simulink model "warplab_mimo_4x4"  (Simulink 6.5)
settings: Solver=ode45  StartTime=0.0  StopTime=20000  RelTol=1e-3
undefined symbols (not defined in the file): gcbh, xlBlockLoadCallback
libraries: xbsIndex_r4 x188
(part 10 of 17)

== system warplab_mimo_4x4/Mem_Control/S-R_Latch (Reverse) ==
  S : Inport
  R : Inport  Port=2
  Convert : S-Function  LoadFcn=xlBlockLoadCallback(gcbh);  FunctionName=sysgen  Parameters=ptable_  mask(Xilinx Type Converter Block){infoedit=Hardware notes: rounding and saturating require hardware resources; truncating and wrapping do not., arith_type_sgadvanced=, arith_type=Boolean, n_bits=16, bin_pt=14, quantization_sgadvanced=, quantization=Truncate, overflow_sgadvanced=, overflow=Wrap, latency=0, dbl_ovrd_sgadvanced=, dbl_ovrd=off, pipeline_sgadvanced=, pipeline=off, xl_use_area_sgadvanced=, xl_use_area=off, xl_area=[0,0,0,0,0,0,0], has_advanced_control=0, sggui_pos=20,20,374,375, block_type=convert, block_version=8.2, sg_icon_stat=30,14,1,1,white,blue,0,0eb6e735, sg_mask_display=|, sg_list_contents=, sg_blockgui_xml=}
      mask sg_mask_display=|
      | fprintf('','COMMENT: begin icon graphics');
      | patch([0 30 30 0 ],[0 0 14 14 ],[0.77 0.82 0.91]);
      | patch([11 9 12 9 11 15 16 17 21 18 15 13 16 13 15 18 21 17 16 15 11 ],[2 4 7 10 12 12 11 12 12 9 12 10 7 4 2 5 2 2 3 2 2 ],[0.98 0.96 0.92]);
      | plot([0 0 30 30 0 ],[0 14 14 0 0 ]);
      | fprintf('','COMMENT: end icon graphics');
      | fprintf('','COMMENT: begin icon text');
      | color('black');port_label('output',1,'cast');
      | fprintf('','COMMENT: end icon text');
      mask prompts: infoedit ""; arith_type_sgadvanced ""; arith_type "Type"; n_bits "Number of bits"; bin_pt "Binary point"; quantization_sgadvanced ""; overflow_sgadvanced ""; dbl_ovrd_sgadvanced ""; dbl_ovrd "Override with doubles"; pipeline_sgadvanced ""; pipeline "Pipeline for maximum performance"; xl_use_area_sgadvanced ""; xl_use_area "Define FPGA area for resource estimation"; xl_area "FPGA area [slices, FFs, BRAMs, LUTs, IOBs, emb. mults, TBUFs]"; has_advanced_control ""; sggui_pos ""; block_type ""; block_version ""; sg_icon_stat ""; sg_mask_display ""; sg_list_contents ""; sg_blockgui_xml ""
      mask help: Hardware notes: rounding and saturating require hardware resources; truncating and wrapping do not.
      mask init: same as warplab_mimo_4x4/Mem_Control/Convert1
      settings: CopyFcn=xlBlockMoveCallback(gcbh);  DeleteFcn=xlDestroyGui(gcbh);  ModelCloseFcn=xlDestroyGui(gcbh);  PreSaveFcn=xlBlockPreSaveCallback(gcbh);  PostSaveFcn=xlBlockPostSaveCallback(gcbh);  DestroyFcn=xlDestroyGui(gcbh);  OpenFcn=xlOpenGui(gcbh, 'convert_gui.xml', @convertenablement, -1)  CloseFcn=xlDestroyGui(gcbh);  MoveFcn=xlBlockMoveCallback(gcbh);
      mask Help: eval('xlWeb(xlhtmldoclink(''Convert''))');
      mask StyleString: edit,edit,popup(Boolean|Signed  (2's comp)|Unsigned),edit,edit,edit,popup(Truncate|Round  (unbiased: +/- Inf)|Round  (unbiased: Even Values)),edit,popup(Wrap|Saturate|Flag as error),edit,edit,checkbox,edit,checkbox,edit,checkbox,edit,edit,edit,edit,edit,edit,edit,edit,edit
      mask Display:
      | fprintf('','COMMENT: begin icon graphics');
      | patch([0 30 30 0 ],[0 0 14 14 ],[0.77 0.82 0.91]);
      | patch([11 9 12 9 11 15 16 17 21 18 15 13 16 13 15 18 21 17 16 15 11 ],[2 4 7 10 12 12 11 12 12 9 12 10 7 4 2 5 2 2 3 2 2 ],[0.98 0.96 0.92]);
      | plot([0 0 30 30 0 ],[0 14 14 0 0 ]);
      | fprintf('','COMMENT: end icon graphics');
      | fprintf('','COMMENT: begin icon text');
      | color('black');port_label('output',1,'cast');
      | fprintf('','COMMENT: end icon text');
  Convert1 : S-Function  LoadFcn=xlBlockLoadCallback(gcbh);  FunctionName=sysgen  Parameters=ptable_  mask(Xilinx Type Converter Block){infoedit=Hardware notes: rounding and saturating require hardware resources; truncating and wrapping do not., arith_type_sgadvanced=, arith_type=Boolean, n_bits=16, bin_pt=14, quantization_sgadvanced=, quantization=Truncate, overflow_sgadvanced=, overflow=Wrap, latency=0, dbl_ovrd_sgadvanced=, dbl_ovrd=off, pipeline_sgadvanced=, pipeline=off, xl_use_area_sgadvanced=, xl_use_area=off, xl_area=[0,0,0,0,0,0,0], has_advanced_control=0, sggui_pos=20,20,374,375, block_type=convert, block_version=8.2, sg_icon_stat=30,14,1,1,white,blue,0,0eb6e735, sg_mask_display=|, sg_list_contents=, sg_blockgui_xml=}
      mask sg_mask_display=|
      | fprintf('','COMMENT: begin icon graphics');
      | patch([0 30 30 0 ],[0 0 14 14 ],[0.77 0.82 0.91]);
      | patch([11 9 12 9 11 15 16 17 21 18 15 13 16 13 15 18 21 17 16 15 11 ],[2 4 7 10 12 12 11 12 12 9 12 10 7 4 2 5 2 2 3 2 2 ],[0.98 0.96 0.92]);
      | plot([0 0 30 30 0 ],[0 14 14 0 0 ]);
      | fprintf('','COMMENT: end icon graphics');
      | fprintf('','COMMENT: begin icon text');
      | color('black');port_label('output',1,'cast');
      | fprintf('','COMMENT: end icon text');
      mask prompts: infoedit ""; arith_type_sgadvanced ""; arith_type "Type"; n_bits "Number of bits"; bin_pt "Binary point"; quantization_sgadvanced ""; overflow_sgadvanced ""; dbl_ovrd_sgadvanced ""; dbl_ovrd "Override with doubles"; pipeline_sgadvanced ""; pipeline "Pipeline for maximum performance"; xl_use_area_sgadvanced ""; xl_use_area "Define FPGA area for resource estimation"; xl_area "FPGA area [slices, FFs, BRAMs, LUTs, IOBs, emb. mults, TBUFs]"; has_advanced_control ""; sggui_pos ""; block_type ""; block_version ""; sg_icon_stat ""; sg_mask_display ""; sg_list_contents ""; sg_blockgui_xml ""
      mask help: Hardware notes: rounding and saturating require hardware resources; truncating and wrapping do not.
      mask init: same as warplab_mimo_4x4/Mem_Control/Convert1
      settings: CopyFcn=xlBlockMoveCallback(gcbh);  DeleteFcn=xlDestroyGui(gcbh);  ModelCloseFcn=xlDestroyGui(gcbh);  PreSaveFcn=xlBlockPreSaveCallback(gcbh);  PostSaveFcn=xlBlockPostSaveCallback(gcbh);  DestroyFcn=xlDestroyGui(gcbh);  OpenFcn=xlOpenGui(gcbh, 'convert_gui.xml', @convertenablement, -1)  CloseFcn=xlDestroyGui(gcbh);  MoveFcn=xlBlockMoveCallback(gcbh);
      mask Help: eval('xlWeb(xlhtmldoclink(''Convert''))');
      mask StyleString: edit,edit,popup(Boolean|Signed  (2's comp)|Unsigned),edit,edit,edit,popup(Truncate|Round  (unbiased: +/- Inf)|Round  (unbiased: Even Values)),edit,popup(Wrap|Saturate|Flag as error),edit,edit,checkbox,edit,checkbox,edit,checkbox,edit,edit,edit,edit,edit,edit,edit,edit,edit
      mask Display:
      | fprintf('','COMMENT: begin icon graphics');
      | patch([0 30 30 0 ],[0 0 14 14 ],[0.77 0.82 0.91]);
      | patch([11 9 12 9 11 15 16 17 21 18 15 13 16 13 15 18 21 17 16 15 11 ],[2 4 7 10 12 12 11 12 12 9 12 10 7 4 2 5 2 2 3 2 2 ],[0.98 0.96 0.92]);
      | plot([0 0 30 30 0 ],[0 14 14 0 0 ]);
      | fprintf('','COMMENT: end icon graphics');
      | fprintf('','COMMENT: begin icon text');
      | color('black');port_label('output',1,'cast');
      | fprintf('','COMMENT: end icon text');
  Register : S-Function  LoadFcn=xlBlockLoadCallback(gcbh);  FunctionName=sysgen  Parameters=ptable_  mask(Xilinx Register Block){init=1, rst_sgadvanced=, rst=on, en_sgadvanced=, en=on, dbl_ovrd_sgadvanced=, dbl_ovrd=off, xl_use_area_sgadvanced=, xl_use_area=off, xl_area=[0,0,0,0,0,0,0], has_advanced_control=0, sggui_pos=-1,-1,-1,-1, block_type=register, block_version=8.2, sg_icon_stat=50,64,3,1,white,blue,0,923c1847, sg_mask_display=|, sg_list_contents=, sg_blockgui_xml=}
      mask sg_mask_display=|
      | fprintf('','COMMENT: begin icon graphics');
      | patch([0 50 50 0 ],[0 0 64 64 ],[0.77 0.82 0.91]);
      | patch([11 3 15 3 11 24 28 32 46 35 24 16 28 16 24 35 46 32 28 24 11 ],[12 20 32 44 52 52 48 52 52 41 52 44 32 20 12 23 12 12 16 12 12 ],[0.98 0.96 0.92]);
      | plot([0 0 50 50 0 ],[0 64 64 0 0 ]);
      | fprintf('','COMMENT: end icon graphics');
      | fprintf('','COMMENT: begin icon text');
      | color('black');port_label('input',1,'d');
      | color('black');port_label('input',2,'rst');
      | color('black');port_label('input',3,'en');
      | color('black');port_label('output',1,'q');
      | color('black');disp('\bf{z^{-1}}','texmode','on');
      | fprintf('','COMMENT: end icon text');
      mask prompts: init "Initial value"; rst_sgadvanced ""; rst "Provide synchronous reset port"; en_sgadvanced ""; en "Provide enable port"; dbl_ovrd_sgadvanced ""; dbl_ovrd "Override with doubles"; xl_use_area_sgadvanced ""; xl_use_area "Define FPGA area for resource estimation"; xl_area "FPGA area [slices, FFs, BRAMs, LUTs, IOBs, emb. mults, TBUFs]"; has_advanced_control ""; sggui_pos ""; block_type ""; block_version ""; sg_icon_stat ""; sg_mask_display ""; sg_list_contents ""; sg_blockgui_xml ""
      mask help: Xilinx Register
      mask init: same as warplab_mimo_4x4/Mem_Control/Register
      settings: CopyFcn=xlBlockMoveCallback(gcbh);  DeleteFcn=xlDestroyGui(gcbh);  ModelCloseFcn=xlDestroyGui(gcbh);  PreSaveFcn=xlBlockPreSaveCallback(gcbh);  PostSaveFcn=xlBlockPostSaveCallback(gcbh);  DestroyFcn=xlDestroyGui(gcbh);  OpenFcn=xlOpenGui(gcbh, 'register_gui.xml', @xlmagicenablement, -1)  CloseFcn=xlDestroyGui(gcbh);  MoveFcn=xlBlockMoveCallback(gcbh);
      mask Help: eval('xlWeb(xlhtmldoclink(''Register''))');
      mask Display:
      | fprintf('','COMMENT: begin icon graphics');
      | patch([0 50 50 0 ],[0 0 64 64 ],[0.77 0.82 0.91]);
      | patch([11 3 15 3 11 24 28 32 46 35 24 16 28 16 24 35 46 32 28 24 11 ],[12 20 32 44 52 52 48 52 52 41 52 44 32 20 12 23 12 12 16 12 12 ],[0.98 0.96 0.92]);
      | plot([0 0 50 50 0 ],[0 64 64 0 0 ]);
      | fprintf('','COMMENT: end icon graphics');
      | fprintf('','COMMENT: begin icon text');
      | color('black');port_label('input',1,'d');
      | color('black');port_label('input',2,'rst');
      | color('black');port_label('input',3,'en');
      | color('black');port_label('output',1,'q');
      | color('black');disp('\bf{z^{-1}}','texmode','on');
      | fprintf('','COMMENT: end icon text');
  zero3 : S-Function  LoadFcn=xlBlockLoadCallback(gcbh);  FunctionName=sysgen  Parameters=ptable_  mask(Xilinx Constant Block Block){arith_type_sgadvanced=, arith_type=Boolean, const=0, n_bits=1, bin_pt=0, explicit_period_sgadvanced=, explicit_period=off, period=1, dsp48_infoedit=The use of this block for DSP48 instructions is deprecated.  Please use the Opmode block., equ=P=C, opselect_sgadvanced=, opselect=C, inp2_sgadvanced=, inp2=PCIN>>17, opr_sgadvanced=, opr=+, inp1_sgadvanced=, inp1=P, carry_sgadvanced=, carry=CIN, dbl_ovrd_sgadvanced=, dbl_ovrd=off, has_advanced_control=0, sggui_pos=-1,-1,-1,-1, block_type=constant, block_version=VER_STRING_GOES_HERE, sg_icon_stat=20,18,0,1,white,blue,0,c7c04a0c, sg_mask_display=|, sg_list_contents=, sg_blockgui_xml=}
      mask sg_mask_display=|
      | fprintf('','COMMENT: begin icon graphics');
      | patch([0 55 55 0 ],[0 0 26 26 ],[0.77 0.82 0.91]);
      | patch([20 16 22 16 20 27 29 31 38 32 26 22 28 22 26 32 38 31 29 27 20 ],[3 7 13 19 23 23 21 23 23 17 23 19 13 7 3 9 3 3 5 3 3 ],[0.98 0.96 0.92]);
      | plot([0 0 55 55 0 ],[0 26 26 0 0 ]);
      | fprintf('','COMMENT: end icon graphics');
      | fprintf('','COMMENT: begin icon text');
      | color('black');port_label('output',1,'0');
      | fprintf('','COMMENT: end icon text');
      mask prompts: arith_type_sgadvanced ""; arith_type "Type"; const "Constant value"; n_bits "Number of bits"; bin_pt "Binary point"; explicit_period_sgadvanced ""; explicit_period "Sampled constant"; period "Sample period"; dsp48_infoedit ""; equ "DSP48 operation"; opselect_sgadvanced ""; opselect "Operation select"; inp2_sgadvanced ""; inp2 "Z mux"; opr_sgadvanced ""; opr "Operand"; inp1_sgadvanced ""; inp1 "YX muxes"; carry_sgadvanced ""; carry "Carry input"; dbl_ovrd_sgadvanced ""; dbl_ovrd "Override with doubles"; has_advanced_control ""; sggui_pos ""; block_type ""; block_version ""; sg_icon_stat ""; sg_mask_display ""; sg_list_contents ""; sg_blockgui_xml ""
      mask help: Xilinx Constant Block
      mask init: same as warplab_mimo_4x4/CaptureDone/zero3
      settings: CopyFcn=xlBlockMoveCallback(gcbh);  DeleteFcn=xlDestroyGui(gcbh);  ModelCloseFcn=xlDestroyGui(gcbh);  PreSaveFcn=xlBlockPreSaveCallback(gcbh);  PostSaveFcn=xlBlockPostSaveCallback(gcbh);  DestroyFcn=xlDestroyGui(gcbh);  OpenFcn=xlOpenGui(gcbh, 'constant_gui.xml', @constantenablement, @constantaction)  CloseFcn=xlDestroyGui(gcbh);  MoveFcn=xlBlockMoveCallback(gcbh);
      mask Help: eval('xlWeb(xlhtmldoclink(''Constant''))');
      mask StyleString: edit,popup(Boolean|Signed (2's comp)|Unsigned|DSP48 Instruction),edit,edit,edit,edit,checkbox,edit,edit,edit,edit,popup(C + A*B|PCIN + A*B|P + A*B|A * B|C + A:B|C - A:B|C|Custom),edit,popup(0|PCIN|P|C|PCIN>>17|P>>17),edit,popup(+|-),edit,popup(0|P|A:B|A*B|C|P+C|A:B+C),edit,popup(0|1|CIN|~SIGN(P or PCIN)|~SIGN(A*B or A:B)|~SIGND(A*B or A:B)),edit,checkbox,edit,edit,edit,edit,edit,edit,edit,edit
      mask Display:
      | fprintf('','COMMENT: begin icon graphics');
      | patch([0 55 55 0 ],[0 0 26 26 ],[0.77 0.82 0.91]);
      | patch([20 16 22 16 20 27 29 31 38 32 26 22 28 22 26 32 38 31 29 27 20 ],[3 7 13 19 23 23 21 23 23 17 23 19 13 7 3 9 3 3 5 3 3 ],[0.98 0.96 0.92]);
      | plot([0 0 55 55 0 ],[0 26 26 0 0 ]);
      | fprintf('','COMMENT: end icon graphics');
      | fprintf('','COMMENT: begin icon text');
      | color('black');port_label('output',1,'0');
      | fprintf('','COMMENT: end icon text');
  Q : Outport
  wires:
  zero3/1 -> Register/1
  S/1 -> Convert/1
  R/1 -> Convert1/1
  Register/1 -> Q/1
  Convert/1 -> Register/2
  Convert1/1 -> Register/3

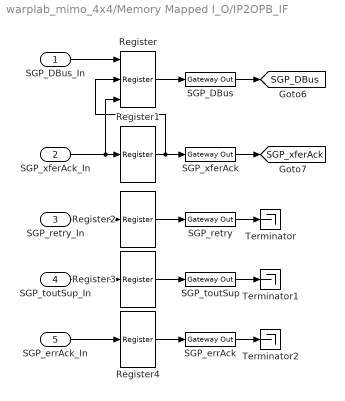
== system warplab_mimo_4x4/Memory Mapped I_O/IP2OPB_IF ==
  SGP_DBus_In : Inport
  SGP_xferAck_In : Inport  Port=2
  SGP_retry_In : Inport  Port=3
  SGP_toutSup_In : Inport  Port=4
  SGP_errAck_In : Inport  Port=5
  Register : xbsIndex_r4/Register  init=0  rst=on  en=on  dbl_ovrd=off  block_type=register
      settings: xl_area=[0, 0, 0, 0, 0, 0, 0]  block_version=VER_STRING_GOES_HERE
  Register{1..4} (4 alike) : xbsIndex_r4/Register  init=0  rst=off  en=off  dbl_ovrd=off  block_type=register
      settings: xl_area=[0, 0, 0, 0, 0, 0, 0]  block_version=VER_STRING_GOES_HERE
  SGP_DBus : xbsIndex_r4/Gateway Out  hdl_port=on  timing_constraint=None  locs_specified=off  LOCs={}  block_type=gatewayout
      settings: infoedit="Gateway out block.  Converts Xilinx fixed point inputs into ouputs of type Simulink integer, double, or fixed point.<P><P>Hardware notes:  In hardware these blocks become top level output ports or are discarded, depending on how they are configured."  xl_area=[0, 0, 0, 0, 0, 0, 0]  block_version=VER_STRING_GOES_HERE
  SGP_errAck : xbsIndex_r4/Gateway Out  hdl_port=on  timing_constraint=None  locs_specified=off  LOCs={}  block_type=gatewayout
      settings: infoedit="Gateway out block.  Converts Xilinx fixed point inputs into ouputs of type Simulink integer, double, or fixed point.<P><P>Hardware notes:  In hardware these blocks become top level output ports or are discarded, depending on how they are configured."  xl_area=[0, 0, 0, 0, 0, 0, 0]  block_version=VER_STRING_GOES_HERE
  SGP_retry : xbsIndex_r4/Gateway Out  hdl_port=on  timing_constraint=None  locs_specified=off  LOCs={}  block_type=gatewayout
      settings: infoedit="Gateway out block.  Converts Xilinx fixed point inputs into ouputs of type Simulink integer, double, or fixed point.<P><P>Hardware notes:  In hardware these blocks become top level output ports or are discarded, depending on how they are configured."  xl_area=[0, 0, 0, 0, 0, 0, 0]  block_version=VER_STRING_GOES_HERE
  SGP_toutSup : xbsIndex_r4/Gateway Out  hdl_port=on  timing_constraint=None  locs_specified=off  LOCs={}  block_type=gatewayout
      settings: infoedit="Gateway out block.  Converts Xilinx fixed point inputs into ouputs of type Simulink integer, double, or fixed point.<P><P>Hardware notes:  In hardware these blocks become top level output ports or are discarded, depending on how they are configured."  xl_area=[0, 0, 0, 0, 0, 0, 0]  block_version=VER_STRING_GOES_HERE
  SGP_xferAck : xbsIndex_r4/Gateway Out  hdl_port=on  timing_constraint=None  locs_specified=off  LOCs={}  block_type=gatewayout
      settings: infoedit="Gateway out block.  Converts Xilinx fixed point inputs into ouputs of type Simulink integer, double, or fixed point.<P><P>Hardware notes:  In hardware these blocks become top level output ports or are discarded, depending on how they are configured."  xl_area=[0, 0, 0, 0, 0, 0, 0]  block_version=VER_STRING_GOES_HERE
  Terminator : Terminator
  Terminator1 : Terminator
  Terminator2 : Terminator
  tag scope: SGP_DBus=global, SGP_xferAck=global
  wires:
  SGP_errAck/1 -> Terminator2/1
  SGP_toutSup/1 -> Terminator1/1
  SGP_retry/1 -> Terminator/1
  Register1/1 -> Register/2, SGP_xferAck/1
  SGP_errAck_In/1 -> Register4/1
  SGP_toutSup_In/1 -> Register3/1
  SGP_retry_In/1 -> Register2/1
  SGP_xferAck_In/1 -> Register1/1, Register/3
  SGP_DBus_In/1 -> Register/1
  SGP_DBus/1 -> [SGP_DBus]
  SGP_xferAck/1 -> [SGP_xferAck]
  Register2/1 -> SGP_retry/1
  Register3/1 -> SGP_toutSup/1
  Register4/1 -> SGP_errAck/1
  Register/1 -> SGP_DBus/1

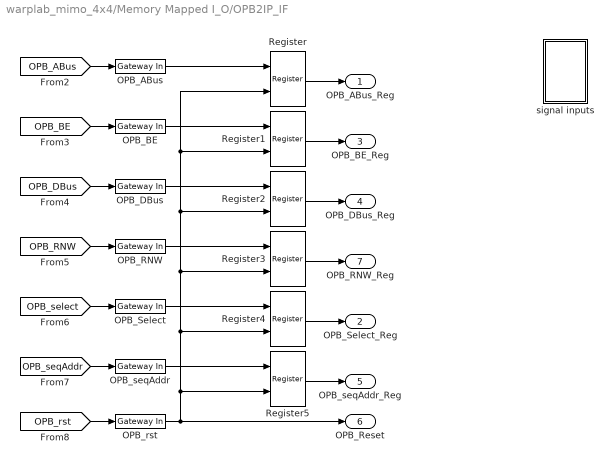
== system warplab_mimo_4x4/Memory Mapped I_O/OPB2IP_IF ==
  OPB_ABus : xbsIndex_r4/Gateway In  arith_type=Unsigned  n_bits=32  bin_pt=0  quantization="Round  (unbiased: +/- Inf)"  overflow=Saturate  period=1  dbl_ovrd=off  timing_constraint=None  locs_specified=off  LOCs={}  block_type=gatewayin
      settings: infoedit="Gateway in block.  Converts inputs of type Simulink integer, double and fixed point to  Xilinx fixed point type.<P><P>Hardware notes:  In hardware these blocks become top level input ports."  xl_area=[0, 0, 0, 0, 0, 0, 0]  block_version=VER_STRING_GOES_HERE
  OPB_BE : xbsIndex_r4/Gateway In  arith_type=Unsigned  n_bits=4  bin_pt=0  quantization="Round  (unbiased: +/- Inf)"  overflow=Saturate  period=1  dbl_ovrd=off  timing_constraint=None  locs_specified=off  LOCs={}  block_type=gatewayin
      settings: infoedit="Gateway in block.  Converts inputs of type Simulink integer, double and fixed point to  Xilinx fixed point type.<P><P>Hardware notes:  In hardware these blocks become top level input ports."  xl_area=[0, 0, 0, 0, 0, 0, 0]  block_version=VER_STRING_GOES_HERE
  OPB_DBus : xbsIndex_r4/Gateway In  arith_type=Unsigned  n_bits=32  bin_pt=0  quantization="Round  (unbiased: +/- Inf)"  overflow=Saturate  period=1  dbl_ovrd=off  timing_constraint=None  locs_specified=off  LOCs={}  block_type=gatewayin
      settings: infoedit="Gateway in block.  Converts inputs of type Simulink integer, double and fixed point to  Xilinx fixed point type.<P><P>Hardware notes:  In hardware these blocks become top level input ports."  xl_area=[0, 0, 0, 0, 0, 0, 0]  block_version=VER_STRING_GOES_HERE
  OPB_RNW : xbsIndex_r4/Gateway In  arith_type=Boolean  n_bits=1  bin_pt=0  quantization="Round  (unbiased: +/- Inf)"  overflow=Saturate  period=1  dbl_ovrd=off  timing_constraint=None  locs_specified=off  LOCs={}  block_type=gatewayin
      settings: infoedit="Gateway in block.  Converts inputs of type Simulink integer, double and fixed point to  Xilinx fixed point type.<P><P>Hardware notes:  In hardware these blocks become top level input ports."  xl_area=[0, 0, 0, 0, 0, 0, 0]  block_version=VER_STRING_GOES_HERE
  OPB_Select : xbsIndex_r4/Gateway In  arith_type=Boolean  n_bits=1  bin_pt=0  quantization="Round  (unbiased: +/- Inf)"  overflow=Saturate  period=1  dbl_ovrd=off  timing_constraint=None  locs_specified=off  LOCs={}  block_type=gatewayin
      settings: infoedit="Gateway in block.  Converts inputs of type Simulink integer, double and fixed point to  Xilinx fixed point type.<P><P>Hardware notes:  In hardware these blocks become top level input ports."  xl_area=[0, 0, 0, 0, 0, 0, 0]  block_version=VER_STRING_GOES_HERE
  OPB_rst : xbsIndex_r4/Gateway In  arith_type=Boolean  n_bits=1  bin_pt=0  quantization="Round  (unbiased: +/- Inf)"  overflow=Saturate  period=1  dbl_ovrd=off  timing_constraint=None  locs_specified=off  LOCs={}  block_type=gatewayin
      settings: infoedit="Gateway in block.  Converts inputs of type Simulink integer, double and fixed point to  Xilinx fixed point type.<P><P>Hardware notes:  In hardware these blocks become top level input ports."  xl_area=[0, 0, 0, 0, 0, 0, 0]  block_version=VER_STRING_GOES_HERE
  OPB_seqAddr : xbsIndex_r4/Gateway In  arith_type=Boolean  n_bits=1  bin_pt=0  quantization="Round  (unbiased: +/- Inf)"  overflow=Saturate  period=1  dbl_ovrd=off  timing_constraint=None  locs_specified=off  LOCs={}  block_type=gatewayin
      settings: infoedit="Gateway in block.  Converts inputs of type Simulink integer, double and fixed point to  Xilinx fixed point type.<P><P>Hardware notes:  In hardware these blocks become top level input ports."  xl_area=[0, 0, 0, 0, 0, 0, 0]  block_version=VER_STRING_GOES_HERE
  Register{,1..5} (6 alike) : xbsIndex_r4/Register  init=0  rst=on  en=off  dbl_ovrd=off  block_type=register
      settings: xl_area=[0, 0, 0, 0, 0, 0, 0]  block_version=VER_STRING_GOES_HERE
  signal inputs : Subsystem
  OPB_ABus_Reg : Outport
  OPB_Select_Reg : Outport  Port=2
  OPB_BE_Reg : Outport  Port=3
  OPB_DBus_Reg : Outport  Port=4
  OPB_seqAddr_Reg : Outport  Port=5
  OPB_Reset : Outport  Port=6
  OPB_RNW_Reg : Outport  Port=7
  wires:
  Register4/1 -> OPB_Select_Reg/1
  OPB_Select/1 -> Register4/1
  OPB_BE/1 -> Register1/1
  OPB_ABus/1 -> Register/1
  [OPB_select] -> OPB_Select/1
  [OPB_seqAddr] -> OPB_seqAddr/1
  [OPB_rst] -> OPB_rst/1
  [OPB_RNW] -> OPB_RNW/1
  [OPB_DBus] -> OPB_DBus/1
  [OPB_BE] -> OPB_BE/1
  [OPB_ABus] -> OPB_ABus/1
  Register/1 -> OPB_ABus_Reg/1
  OPB_rst/1 -> Register4/2, Register1/2, Register/2, Register2/2, Register3/2, Register5/2, OPB_Reset/1
  Register5/1 -> OPB_seqAddr_Reg/1
  Register3/1 -> OPB_RNW_Reg/1
  Register2/1 -> OPB_DBus_Reg/1
  Register1/1 -> OPB_BE_Reg/1
  OPB_seqAddr/1 -> Register5/1
  OPB_RNW/1 -> Register3/1
  OPB_DBus/1 -> Register2/1

== system warplab_mimo_4x4/Memory Mapped I_O/ack_gen ==
  ps : Inport
  rst : Inport  Port=2
  Inverter1 : xbsIndex_r4/Inverter  en=off  latency=0  dbl_ovrd=off  block_type=inv
      settings: xl_area=[0, 0, 0, 0, 0, 0, 0]  block_version=VER_STRING_GOES_HERE
  Inverter2 : xbsIndex_r4/Inverter  en=off  latency=0  dbl_ovrd=off  block_type=inv
      settings: xl_area=[0, 0, 0, 0, 0, 0, 0]  block_version=VER_STRING_GOES_HERE
  Logical : xbsIndex_r4/Logical  logical_function=AND  inputs=3  en=off  latency=0  precision=Full  arith_type=Unsigned  n_bits=8  bin_pt=2  align_bp=on  dbl_ovrd=off  block_type=logical
      settings: xl_area=[0, 0, 0, 0, 0, 0, 0]  block_version=VER_STRING_GOES_HERE
  Register : xbsIndex_r4/Register  init=0  rst=off  en=off  dbl_ovrd=off  block_type=register
      settings: xl_area=[0, 0, 0, 0, 0, 0, 0]  block_version=VER_STRING_GOES_HERE
  ack : Outport
  wires:
  Logical/1 -> ack/1
  rst/1 -> Inverter1/1
  Inverter1/1 -> Logical/3
  Register/1 -> Inverter2/1
  Inverter2/1 -> Logical/2
  ps/1 -> Register/1, Logical/1

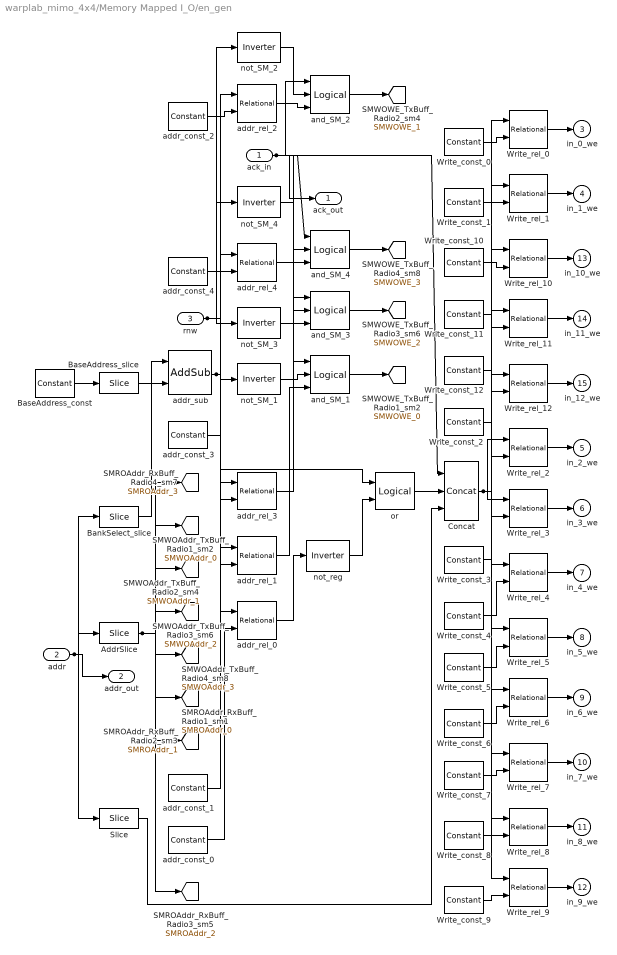
== system warplab_mimo_4x4/Memory Mapped I_O/en_gen ==
  ack_in : Inport
  addr : Inport  Port=2
  rnw : Inport  Port=3
  AddrSlice : xbsIndex_r4/Slice  nbits=14  boolean_output=off  mode=Lower Bit Location + Width  bit1=0  base1=MSB of Input  bit0=2  base0=LSB of Input  dbl_ovrd=off  block_type=slice
      settings: infoedit="Extracts a given range of bits from each input sample and presents it at the output.  The output type is ordinarily unsigned with binary point at zero, but can be Boolean when the slice is one bit wide.<P><P>Hardware notes: In hardware this block costs nothing."  block_version=VER_STRING_GOES_HERE
  BankSelect_slice : xbsIndex_r4/Slice  nbits=4  boolean_output=off  mode=Lower Bit Location + Width  bit1=0  base1=MSB of Input  bit0=16  base0=LSB of Input  dbl_ovrd=off  block_type=slice
      settings: infoedit="Extracts a given range of bits from each input sample and presents it at the output.  The output type is ordinarily unsigned with binary point at zero, but can be Boolean when the slice is one bit wide.<P><P>Hardware notes: In hardware this block costs nothing."  block_version=VER_STRING_GOES_HERE
  BaseAddress_const : xbsIndex_r4/Constant  arith_type=Unsigned  const=0  n_bits=32  bin_pt=0  explicit_period=off  period=1  equ=P=C  opselect=C  inp2=PCIN>>17  opr=+  inp1=P  carry=CIN  dbl_ovrd=off  block_type=constant
      settings: block_version=VER_STRING_GOES_HERE
  BaseAddress_slice : xbsIndex_r4/Slice  nbits=4  boolean_output=off  mode=Lower Bit Location + Width  bit1=0  base1=MSB of Input  bit0=16  base0=LSB of Input  dbl_ovrd=off  block_type=slice
      settings: infoedit="Extracts a given range of bits from each input sample and presents it at the output.  The output type is ordinarily unsigned with binary point at zero, but can be Boolean when the slice is one bit wide.<P><P>Hardware notes: In hardware this block costs nothing."  block_version=VER_STRING_GOES_HERE
  Concat : xbsIndex_r4/Concat  num_inputs=3  dbl_ovrd=off  block_type=concat
      settings: block_version=VER_STRING_GOES_HERE
  Slice : xbsIndex_r4/Slice  nbits=4  boolean_output=off  mode=Lower Bit Location + Width  bit1=0  base1=MSB of Input  bit0=2  base0=LSB of Input  dbl_ovrd=off  block_type=slice
      settings: infoedit="Extracts a given range of bits from each input sample and presents it at the output.  The output type is ordinarily unsigned with binary point at zero, but can be Boolean when the slice is one bit wide.<P><P>Hardware notes: In hardware this block costs nothing."  block_version=VER_STRING_GOES_HERE
  Write_const_0 : xbsIndex_r4/Constant  arith_type=Unsigned  const=32  n_bits=6  bin_pt=0  explicit_period=off  period=1  equ=P=C  opselect=C  inp2=PCIN>>17  opr=+  inp1=P  carry=CIN  dbl_ovrd=off  block_type=constant
      settings: block_version=VER_STRING_GOES_HERE
  Write_const_1 : xbsIndex_r4/Constant  arith_type=Unsigned  const=33  n_bits=6  bin_pt=0  explicit_period=off  period=1  equ=P=C  opselect=C  inp2=PCIN>>17  opr=+  inp1=P  carry=CIN  dbl_ovrd=off  block_type=constant
      settings: block_version=VER_STRING_GOES_HERE
  Write_const_10 : xbsIndex_r4/Constant  arith_type=Unsigned  const=42  n_bits=6  bin_pt=0  explicit_period=off  period=1  equ=P=C  opselect=C  inp2=PCIN>>17  opr=+  inp1=P  carry=CIN  dbl_ovrd=off  block_type=constant
      settings: block_version=VER_STRING_GOES_HERE
  Write_const_11 : xbsIndex_r4/Constant  arith_type=Unsigned  const=43  n_bits=6  bin_pt=0  explicit_period=off  period=1  equ=P=C  opselect=C  inp2=PCIN>>17  opr=+  inp1=P  carry=CIN  dbl_ovrd=off  block_type=constant
      settings: block_version=VER_STRING_GOES_HERE
  Write_const_12 : xbsIndex_r4/Constant  arith_type=Unsigned  const=44  n_bits=6  bin_pt=0  explicit_period=off  period=1  equ=P=C  opselect=C  inp2=PCIN>>17  opr=+  inp1=P  carry=CIN  dbl_ovrd=off  block_type=constant
      settings: block_version=VER_STRING_GOES_HERE
  Write_const_2 : xbsIndex_r4/Constant  arith_type=Unsigned  const=34  n_bits=6  bin_pt=0  explicit_period=off  period=1  equ=P=C  opselect=C  inp2=PCIN>>17  opr=+  inp1=P  carry=CIN  dbl_ovrd=off  block_type=constant
      settings: block_version=VER_STRING_GOES_HERE
  Write_const_3 : xbsIndex_r4/Constant  arith_type=Unsigned  const=35  n_bits=6  bin_pt=0  explicit_period=off  period=1  equ=P=C  opselect=C  inp2=PCIN>>17  opr=+  inp1=P  carry=CIN  dbl_ovrd=off  block_type=constant
      settings: block_version=VER_STRING_GOES_HERE
  Write_const_4 : xbsIndex_r4/Constant  arith_type=Unsigned  const=36  n_bits=6  bin_pt=0  explicit_period=off  period=1  equ=P=C  opselect=C  inp2=PCIN>>17  opr=+  inp1=P  carry=CIN  dbl_ovrd=off  block_type=constant
      settings: block_version=VER_STRING_GOES_HERE
  Write_const_5 : xbsIndex_r4/Constant  arith_type=Unsigned  const=37  n_bits=6  bin_pt=0  explicit_period=off  period=1  equ=P=C  opselect=C  inp2=PCIN>>17  opr=+  inp1=P  carry=CIN  dbl_ovrd=off  block_type=constant
      settings: block_version=VER_STRING_GOES_HERE
  Write_const_6 : xbsIndex_r4/Constant  arith_type=Unsigned  const=38  n_bits=6  bin_pt=0  explicit_period=off  period=1  equ=P=C  opselect=C  inp2=PCIN>>17  opr=+  inp1=P  carry=CIN  dbl_ovrd=off  block_type=constant
      settings: block_version=VER_STRING_GOES_HERE
  Write_const_7 : xbsIndex_r4/Constant  arith_type=Unsigned  const=39  n_bits=6  bin_pt=0  explicit_period=off  period=1  equ=P=C  opselect=C  inp2=PCIN>>17  opr=+  inp1=P  carry=CIN  dbl_ovrd=off  block_type=constant
      settings: block_version=VER_STRING_GOES_HERE
  Write_const_8 : xbsIndex_r4/Constant  arith_type=Unsigned  const=40  n_bits=6  bin_pt=0  explicit_period=off  period=1  equ=P=C  opselect=C  inp2=PCIN>>17  opr=+  inp1=P  carry=CIN  dbl_ovrd=off  block_type=constant
      settings: block_version=VER_STRING_GOES_HERE
  Write_const_9 : xbsIndex_r4/Constant  arith_type=Unsigned  const=41  n_bits=6  bin_pt=0  explicit_period=off  period=1  equ=P=C  opselect=C  inp2=PCIN>>17  opr=+  inp1=P  carry=CIN  dbl_ovrd=off  block_type=constant
      settings: block_version=VER_STRING_GOES_HERE
  Write_rel_{0..12} (13 alike) : xbsIndex_r4/Relational  mode=a=b  en=off  latency=0  dbl_ovrd=off  block_type=relational
      settings: xl_area=[0, 0, 0, 0, 0, 0, 0]  block_version=VER_STRING_GOES_HERE
  addr_const_0 : xbsIndex_r4/Constant  arith_type=Unsigned  const=0  n_bits=4  bin_pt=0  explicit_period=off  period=1  equ=P=C  opselect=C  inp2=PCIN>>17  opr=+  inp1=P  carry=CIN  dbl_ovrd=off  block_type=constant
      settings: block_version=VER_STRING_GOES_HERE
  addr_const_1 : xbsIndex_r4/Constant  arith_type=Unsigned  const=5  n_bits=4  bin_pt=0  explicit_period=off  period=1  equ=P=C  opselect=C  inp2=PCIN>>17  opr=+  inp1=P  carry=CIN  dbl_ovrd=off  block_type=constant
      settings: block_version=VER_STRING_GOES_HERE
  addr_const_2 : xbsIndex_r4/Constant  arith_type=Unsigned  const=6  n_bits=4  bin_pt=0  explicit_period=off  period=1  equ=P=C  opselect=C  inp2=PCIN>>17  opr=+  inp1=P  carry=CIN  dbl_ovrd=off  block_type=constant
      settings: block_version=VER_STRING_GOES_HERE
  addr_const_3 : xbsIndex_r4/Constant  arith_type=Unsigned  const=7  n_bits=4  bin_pt=0  explicit_period=off  period=1  equ=P=C  opselect=C  inp2=PCIN>>17  opr=+  inp1=P  carry=CIN  dbl_ovrd=off  block_type=constant
      settings: block_version=VER_STRING_GOES_HERE
  addr_const_4 : xbsIndex_r4/Constant  arith_type=Unsigned  const=8  n_bits=4  bin_pt=0  explicit_period=off  period=1  equ=P=C  opselect=C  inp2=PCIN>>17  opr=+  inp1=P  carry=CIN  dbl_ovrd=off  block_type=constant
      settings: block_version=VER_STRING_GOES_HERE
  addr_rel_{0..4} (5 alike) : xbsIndex_r4/Relational  mode=a=b  en=off  latency=0  dbl_ovrd=off  block_type=relational
      settings: xl_area=[0, 0, 0, 0, 0, 0, 0]  block_version=VER_STRING_GOES_HERE
  addr_sub : xbsIndex_r4/AddSub  mode=Subtraction  use_carryin=off  use_carryout=off  en=off  latency=0  precision=User Defined  arith_type=Unsigned  n_bits=4  bin_pt=0  quantization=Truncate  overflow=Wrap  dbl_ovrd=off  use_behavioral_HDL=off  pipelined=off  use_rpm=on  block_type=addsub
      settings: block_version=VER_STRING_GOES_HERE
  and_SM_{1..4} (4 alike) : xbsIndex_r4/Logical  logical_function=AND  inputs=3  en=off  latency=0  precision=Full  arith_type=Unsigned  n_bits=16  bin_pt=0  align_bp=on  dbl_ovrd=off  block_type=logical
      settings: block_version=VER_STRING_GOES_HERE
  not_SM_{1..4} (4 alike) : xbsIndex_r4/Inverter  en=off  latency=0  dbl_ovrd=off  block_type=inv
      settings: block_version=VER_STRING_GOES_HERE
  not_reg : xbsIndex_r4/Inverter  en=off  latency=0  dbl_ovrd=off  block_type=inv
      settings: block_version=VER_STRING_GOES_HERE
  or : xbsIndex_r4/Logical  logical_function=OR  inputs=2  en=off  latency=0  precision=Full  arith_type=Unsigned  n_bits=16  bin_pt=0  align_bp=on  dbl_ovrd=off  block_type=logical
      settings: block_version=VER_STRING_GOES_HERE
  ack_out : Outport
  addr_out : Outport  Port=2
  in_0_we : Outport  Port=3
  in_1_we : Outport  Port=4
  in_2_we : Outport  Port=5
  in_3_we : Outport  Port=6
  in_4_we : Outport  Port=7
  in_5_we : Outport  Port=8
  in_6_we : Outport  Port=9
  in_7_we : Outport  Port=10
  in_8_we : Outport  Port=11
  in_9_we : Outport  Port=12
  in_10_we : Outport  Port=13
  in_11_we : Outport  Port=14
  in_12_we : Outport  Port=15
  tag scope: SMROAddr_0=global, SMROAddr_1=global, SMROAddr_2=global, SMROAddr_3=global, SMWOAddr_0=global, SMWOAddr_1=global, SMWOAddr_2=global, SMWOAddr_3=global, SMWOWE_0=global, SMWOWE_1=global, SMWOWE_2=global, SMWOWE_3=global
  wires:
  ack_in/1 -> and_SM_4/1, and_SM_3/1, and_SM_2/1, and_SM_1/1, Concat/1, ack_out/1
  addr/1 -> BankSelect_slice/1, AddrSlice/1, Slice/1, addr_out/1
  Concat/1 -> Write_rel_12/1, Write_rel_11/1, Write_rel_10/1, Write_rel_9/1, Write_rel_8/1, Write_rel_7/1, Write_rel_6/1, Write_rel_5/1, Write_rel_4/1, Write_rel_3/1, Write_rel_2/1, Write_rel_1/1, Write_rel_0/1
  AddrSlice/1 -> [SMWOAddr_3], [SMWOAddr_2], [SMWOAddr_1], [SMWOAddr_0], [SMROAddr_3], [SMROAddr_2], [SMROAddr_1], [SMROAddr_0]
  addr_sub/1 -> addr_rel_4/1, addr_rel_3/1, addr_rel_2/1, addr_rel_1/1, addr_rel_0/1
  rnw/1 -> not_SM_4/1, not_SM_3/1, not_SM_2/1, not_SM_1/1, or/1
  and_SM_4/1 -> [SMWOWE_3]
  addr_rel_4/1 -> and_SM_4/3
  not_SM_4/1 -> and_SM_4/2
  addr_const_4/1 -> addr_rel_4/2
  and_SM_3/1 -> [SMWOWE_2]
  addr_rel_3/1 -> and_SM_3/3
  not_SM_3/1 -> and_SM_3/2
  addr_const_3/1 -> addr_rel_3/2
  and_SM_2/1 -> [SMWOWE_1]
  addr_rel_2/1 -> and_SM_2/3
  not_SM_2/1 -> and_SM_2/2
  addr_const_2/1 -> addr_rel_2/2
  and_SM_1/1 -> [SMWOWE_0]
  addr_rel_1/1 -> and_SM_1/3
  not_SM_1/1 -> and_SM_1/2
  addr_const_1/1 -> addr_rel_1/2
  or/1 -> Concat/2
  not_reg/1 -> or/2
  addr_rel_0/1 -> not_reg/1
  addr_const_0/1 -> addr_rel_0/2
  BaseAddress_slice/1 -> addr_sub/2
  BankSelect_slice/1 -> addr_sub/1
  BaseAddress_const/1 -> BaseAddress_slice/1
  Write_rel_12/1 -> in_12_we/1
  Write_const_12/1 -> Write_rel_12/2
  Write_rel_11/1 -> in_11_we/1
  Write_const_11/1 -> Write_rel_11/2
  Write_rel_10/1 -> in_10_we/1
  Write_const_10/1 -> Write_rel_10/2
  Write_rel_9/1 -> in_9_we/1
  Write_const_9/1 -> Write_rel_9/2
  Write_rel_8/1 -> in_8_we/1
  Write_const_8/1 -> Write_rel_8/2
  Write_rel_7/1 -> in_7_we/1
  Write_const_7/1 -> Write_rel_7/2
  Write_rel_6/1 -> in_6_we/1
  Write_const_6/1 -> Write_rel_6/2
  Write_rel_5/1 -> in_5_we/1
  Write_const_5/1 -> Write_rel_5/2
  Write_rel_4/1 -> in_4_we/1
  Write_const_4/1 -> Write_rel_4/2
  Write_rel_3/1 -> in_3_we/1
  Write_const_3/1 -> Write_rel_3/2
  Write_rel_2/1 -> in_2_we/1
  Write_const_2/1 -> Write_rel_2/2
  Write_rel_1/1 -> in_1_we/1
  Write_const_1/1 -> Write_rel_1/2
  Write_rel_0/1 -> in_0_we/1
  Write_const_0/1 -> Write_rel_0/2
  Slice/1 -> Concat/3

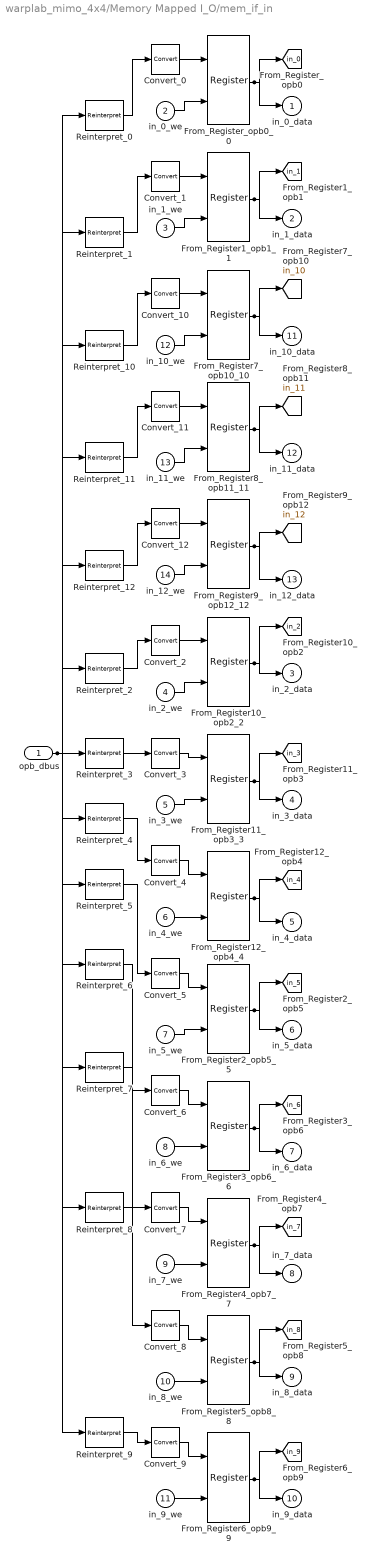
== system warplab_mimo_4x4/Memory Mapped I_O/mem_if_in ==
  opb_dbus : Inport
  in_0_we : Inport  Port=2
  in_1_we : Inport  Port=3
  in_2_we : Inport  Port=4
  in_3_we : Inport  Port=5
  in_4_we : Inport  Port=6
  in_5_we : Inport  Port=7
  in_6_we : Inport  Port=8
  in_7_we : Inport  Port=9
  in_8_we : Inport  Port=10
  in_9_we : Inport  Port=11
  in_10_we : Inport  Port=12
  in_11_we : Inport  Port=13
  in_12_we : Inport  Port=14
  Convert_0 : xbsIndex_r4/Convert  arith_type=Unsigned  n_bits=14  bin_pt=0  quantization=Truncate  overflow=Wrap  latency=0  dbl_ovrd=off  pipeline=off  block_type=convert
      settings: xl_area=[0, 0, 0, 0, 0, 0, 0]  block_version=VER_STRING_GOES_HERE
  Convert_{1..6,8..12} (11 alike) : xbsIndex_r4/Convert  arith_type=Unsigned  n_bits=1  bin_pt=0  quantization=Truncate  overflow=Wrap  latency=0  dbl_ovrd=off  pipeline=off  block_type=convert
      settings: xl_area=[0, 0, 0, 0, 0, 0, 0]  block_version=VER_STRING_GOES_HERE
  Convert_7 : xbsIndex_r4/Convert  arith_type=Unsigned  n_bits=14  bin_pt=0  quantization=Truncate  overflow=Wrap  latency=0  dbl_ovrd=off  pipeline=off  block_type=convert
      settings: xl_area=[0, 0, 0, 0, 0, 0, 0]  block_version=VER_STRING_GOES_HERE
  From_Register10_opb2_2 : xbsIndex_r4/Register  init=0  rst=off  en=on  dbl_ovrd=off  block_type=register
      settings: xl_area=[0, 0, 0, 0, 0, 0, 0]  block_version=VER_STRING_GOES_HERE
  From_Register11_opb3_3 : xbsIndex_r4/Register  init=0  rst=off  en=on  dbl_ovrd=off  block_type=register
      settings: xl_area=[0, 0, 0, 0, 0, 0, 0]  block_version=VER_STRING_GOES_HERE
  From_Register12_opb4_4 : xbsIndex_r4/Register  init=0  rst=off  en=on  dbl_ovrd=off  block_type=register
      settings: xl_area=[0, 0, 0, 0, 0, 0, 0]  block_version=VER_STRING_GOES_HERE
  From_Register1_opb1_1 : xbsIndex_r4/Register  init=0  rst=off  en=on  dbl_ovrd=off  block_type=register
      settings: xl_area=[0, 0, 0, 0, 0, 0, 0]  block_version=VER_STRING_GOES_HERE
  From_Register2_opb5_5 : xbsIndex_r4/Register  init=0  rst=off  en=on  dbl_ovrd=off  block_type=register
      settings: xl_area=[0, 0, 0, 0, 0, 0, 0]  block_version=VER_STRING_GOES_HERE
  From_Register3_opb6_6 : xbsIndex_r4/Register  init=0  rst=off  en=on  dbl_ovrd=off  block_type=register
      settings: xl_area=[0, 0, 0, 0, 0, 0, 0]  block_version=VER_STRING_GOES_HERE
  From_Register4_opb7_7 : xbsIndex_r4/Register  init=2^14-1  rst=off  en=on  dbl_ovrd=off  block_type=register
      settings: xl_area=[0, 0, 0, 0, 0, 0, 0]  block_version=VER_STRING_GOES_HERE
  From_Register5_opb8_8 : xbsIndex_r4/Register  init=0  rst=off  en=on  dbl_ovrd=off  block_type=register
      settings: xl_area=[0, 0, 0, 0, 0, 0, 0]  block_version=VER_STRING_GOES_HERE
  From_Register6_opb9_9 : xbsIndex_r4/Register  init=0  rst=off  en=on  dbl_ovrd=off  block_type=register
      settings: xl_area=[0, 0, 0, 0, 0, 0, 0]  block_version=VER_STRING_GOES_HERE
  From_Register7_opb10_10 : xbsIndex_r4/Register  init=0  rst=off  en=on  dbl_ovrd=off  block_type=register
      settings: xl_area=[0, 0, 0, 0, 0, 0, 0]  block_version=VER_STRING_GOES_HERE
  From_Register8_opb11_11 : xbsIndex_r4/Register  init=0  rst=off  en=on  dbl_ovrd=off  block_type=register
      settings: xl_area=[0, 0, 0, 0, 0, 0, 0]  block_version=VER_STRING_GOES_HERE
  From_Register9_opb12_12 : xbsIndex_r4/Register  init=0  rst=off  en=on  dbl_ovrd=off  block_type=register
      settings: xl_area=[0, 0, 0, 0, 0, 0, 0]  block_version=VER_STRING_GOES_HERE
  From_Register_opb0_0 : xbsIndex_r4/Register  init=100  rst=off  en=on  dbl_ovrd=off  block_type=register
      settings: xl_area=[0, 0, 0, 0, 0, 0, 0]  block_version=VER_STRING_GOES_HERE
  Reinterpret_{0..12} (13 alike) : xbsIndex_r4/Reinterpret  force_arith_type=on  arith_type=Unsigned  force_bin_pt=on  bin_pt=0  block_type=cast
      settings: infoedit="Changes type of samples without altering their binary representation.<P><P>Hardware notes: In hardware this block costs nothing.<P><P>Example:  Suppose the input is 6 bits wide, signed, with 2 fractional bits, and the output is forced to unsigned with 0 fractional bits.  Then an input of -2.0 (1110.00 in binary 2's complement) becomes an output of 56 (111000 in binary)."  block_version=VER_STRING_GOES_HERE
  in_0_data : Outport
  in_1_data : Outport  Port=2
  in_2_data : Outport  Port=3
  in_3_data : Outport  Port=4
  in_4_data : Outport  Port=5
  in_5_data : Outport  Port=6
  in_6_data : Outport  Port=7
  in_7_data : Outport  Port=8
  in_8_data : Outport  Port=9
  in_9_data : Outport  Port=10
  in_10_data : Outport  Port=11
  in_11_data : Outport  Port=12
  in_12_data : Outport  Port=13
  tag scope: in_0=global, in_10=global, in_11=global, in_12=global, in_1=global, in_2=global, in_3=global, in_4=global, in_5=global, in_6=global, in_7=global, in_8=global, in_9=global
  wires:
  From_Register_opb0_0/1 -> in_0_data/1, [in_0]
  opb_dbus/1 -> Reinterpret_12/1, Reinterpret_11/1, Reinterpret_10/1, Reinterpret_9/1, Reinterpret_8/1, Reinterpret_7/1, Reinterpret_6/1, Reinterpret_5/1, Reinterpret_4/1, Reinterpret_3/1, Reinterpret_2/1, Reinterpret_1/1, Reinterpret_0/1
  From_Register1_opb1_1/1 -> in_1_data/1, [in_1]
  From_Register10_opb2_2/1 -> in_2_data/1, [in_2]
  From_Register11_opb3_3/1 -> in_3_data/1, [in_3]
  From_Register12_opb4_4/1 -> in_4_data/1, [in_4]
  From_Register2_opb5_5/1 -> in_5_data/1, [in_5]
  From_Register3_opb6_6/1 -> in_6_data/1, [in_6]
  From_Register4_opb7_7/1 -> in_7_data/1, [in_7]
  From_Register5_opb8_8/1 -> in_8_data/1, [in_8]
  From_Register6_opb9_9/1 -> in_9_data/1, [in_9]
  From_Register7_opb10_10/1 -> in_10_data/1, [in_10]
  From_Register8_opb11_11/1 -> in_11_data/1, [in_11]
  From_Register9_opb12_12/1 -> in_12_data/1, [in_12]
  in_12_we/1 -> From_Register9_opb12_12/2
  Convert_12/1 -> From_Register9_opb12_12/1
  Reinterpret_12/1 -> Convert_12/1
  in_11_we/1 -> From_Register8_opb11_11/2
  Convert_11/1 -> From_Register8_opb11_11/1
  Reinterpret_11/1 -> Convert_11/1
  in_10_we/1 -> From_Register7_opb10_10/2
  Convert_10/1 -> From_Register7_opb10_10/1
  Reinterpret_10/1 -> Convert_10/1
  in_9_we/1 -> From_Register6_opb9_9/2
  Convert_9/1 -> From_Register6_opb9_9/1
  Reinterpret_9/1 -> Convert_9/1
  in_8_we/1 -> From_Register5_opb8_8/2
  Convert_8/1 -> From_Register5_opb8_8/1
  Reinterpret_8/1 -> Convert_8/1
  in_7_we/1 -> From_Register4_opb7_7/2
  Convert_7/1 -> From_Register4_opb7_7/1
  Reinterpret_7/1 -> Convert_7/1
  in_6_we/1 -> From_Register3_opb6_6/2
  Convert_6/1 -> From_Register3_opb6_6/1
  Reinterpret_6/1 -> Convert_6/1
  in_5_we/1 -> From_Register2_opb5_5/2
  Convert_5/1 -> From_Register2_opb5_5/1
  Reinterpret_5/1 -> Convert_5/1
  in_4_we/1 -> From_Register12_opb4_4/2
  Convert_4/1 -> From_Register12_opb4_4/1
  Reinterpret_4/1 -> Convert_4/1
  in_3_we/1 -> From_Register11_opb3_3/2
  Convert_3/1 -> From_Register11_opb3_3/1
  Reinterpret_3/1 -> Convert_3/1
  in_2_we/1 -> From_Register10_opb2_2/2
  Convert_2/1 -> From_Register10_opb2_2/1
  Reinterpret_2/1 -> Convert_2/1
  in_1_we/1 -> From_Register1_opb1_1/2
  Convert_1/1 -> From_Register1_opb1_1/1
  Reinterpret_1/1 -> Convert_1/1
  in_0_we/1 -> From_Register_opb0_0/2
  Convert_0/1 -> From_Register_opb0_0/1
  Reinterpret_0/1 -> Convert_0/1
